simulink model "UKFSIM"  (R2019a)
settings: Solver=VariableStepAuto  StartTime=0.0  StopTime=50000  RelTol=1e-3
values from neighbouring files (symbols this model uses):
  A1 = 5    [run.m]
  A2 = 5    [run.m]
  A3 = 5    [run.m]
libraries: simulink x1
settings Model: Creator=Nima  LastModifiedBy=Nima

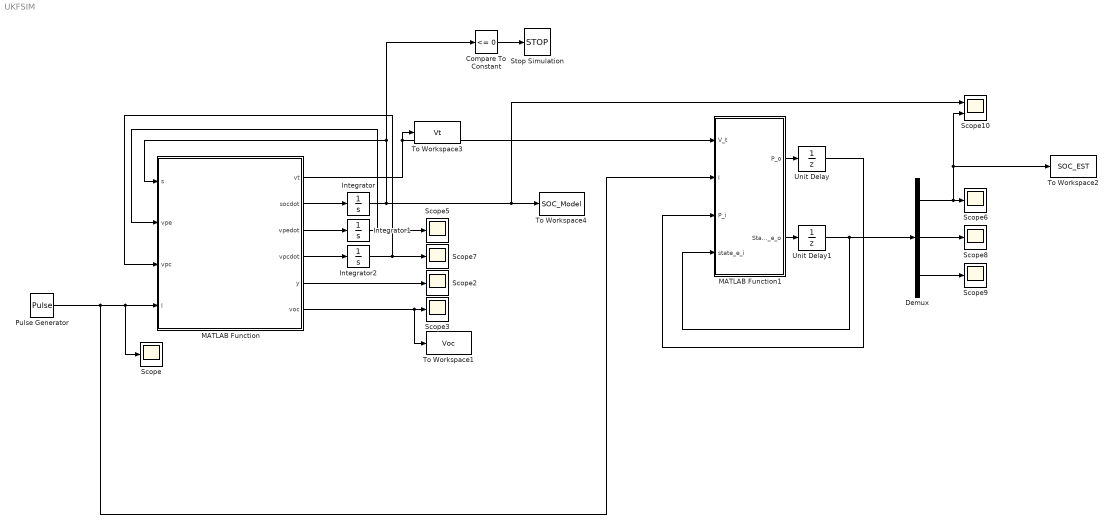
== system UKFSIM ==
  Compare To Constant : simulink/Logic and Bit Operations/Compare To Constant  relop=<=  const=0  OutDataTypeStr=boolean
  Demux : Demux  Outputs=3
  Integrator : Integrator  InitialCondition=1
  Integrator1 : Integrator
  Integrator2 : Integrator
  MATLAB Function : MATLAB Function  TreatAsAtomicUnit=on
  MATLAB Function1 : MATLAB Function  TreatAsAtomicUnit=on
  Pulse Generator : DiscretePulseGenerator  PulseType=Time based  Amplitude=5  Period=5000  PulseWidth=10
  Scope{,2..3,5..9} (8 alike) : Scope
  Scope10 : Scope  NumInputPorts=2
  Stop Simulation : Stop
  To Workspace1 : ToWorkspace  VariableName=Voc  SaveFormat=Timeseries  SampleTime=-1
  To Workspace2 : ToWorkspace  VariableName=SOC_EST  SaveFormat=Timeseries  SampleTime=-1
  To Workspace3 : ToWorkspace  VariableName=Vt  SaveFormat=Timeseries  SampleTime=-1
  To Workspace4 : ToWorkspace  VariableName=SOC_Model  SaveFormat=Timeseries  SampleTime=-1
  Unit Delay : UnitDelay  InitialCondition=diag([A1 A2 A3])  SampleTime=0.01  HasFrameUpgradeWarning=on
  Unit Delay1 : UnitDelay  InitialCondition=[0.2,0,0]  SampleTime=0.01  HasFrameUpgradeWarning=on
  wires:
  MATLAB Function/2(socdot) -> Integrator/1
  MATLAB Function/3(vpedot) -> Integrator1/1
  MATLAB Function/4(vpcdot) -> Integrator2/1
  MATLAB Function/5(y) -> Scope2/1
  MATLAB Function/6(voc) -> To Workspace1/1, Scope3/1
  Integrator1/1 -> MATLAB Function/2(vpe), Scope5/1
  Unit Delay1/1 -> Demux/1, MATLAB Function1/4(state_e_i)
  MATLAB Function/1(vt) -> MATLAB Function1/1(V_t), To Workspace3/1
  MATLAB Function1/1(P_o) -> Unit Delay/1
  MATLAB Function1/2(State_e_o) -> Unit Delay1/1
  Pulse Generator/1 -> MATLAB Function1/2(I), Scope/1, MATLAB Function/4(I)
  Unit Delay/1 -> MATLAB Function1/3(P_i)
  Demux/2 -> Scope8/1
  Demux/1 -> To Workspace2/1, Scope10/2, Scope6/1
  Demux/3 -> Scope9/1
  Compare To Constant/1 -> Stop Simulation/1
  Integrator/1 -> Scope10/1, To Workspace4/1, Compare To Constant/1, MATLAB Function/1(s)
  Integrator2/1 -> MATLAB Function/3(vpc), Scope7/1

== matlab function UKFSIM/MATLAB Function1 ==
  data: V_t input; P_o output; I input; P_i input; state_e_i input; State_e_o output
function [P_o,State_e_o] = fcn(V_t,I,P_i,state_e_i)
%%
%{
sigma_xx(:,k)=[
    sigma_x(1,k)=soc(k-1);
    sigma_x(2,k)=Vpe(k-1);
    sigma_x(3,k)=Vpc(k-1);
]

sigma_xxx(:,i)-->
sigma_xxx(1,k)= soc(k-1);
sigma_xxx(2,k)= Vpe(k-1);
sigma_xxx(3,k)= Vpc(k-1);
sigma_z(1,k)=vt;
%}
%% Battery Parameters
R_pe=4.96e-3;
R_pc=2.86e-3;
C_pe=4.93e3;
C_pc=14.33e3;
R_in=102.5e-3;
C_n=5*3600;
%% 
n=3;
n_m=2*n+1;
kappa=0;
alpha=0.6;
beta=300;
%% 7.34
lambda=alpha^2*(n+kappa)-n;
wm = ones(n_m,1)*1/(2*(n+lambda));
wc = wm;
wm(1)= lambda/(lambda+n); 
wc(1)= lambda/(lambda+n)+1-alpha^2+beta;
sigma_x=zeros(3,n_m);
sigma_xx=zeros(3,n_m);
sigma_xxx=zeros(3,n_m);
sigma_z=zeros(1,n_m);
P_sqrt=chol(P_i,'lower');
%%
% Q = diag([0.02 0.1 0.2]);R=0.2;   
%% 7.39 Calculate sigma point
for i=1:1:n_m
    if i==1
        sigma_x(:,i)= state_e_i;
    elseif i>=2 && i<=n+1
        sigma_x(:,i)= state_e_i+sqrt(n+lambda)*(P_sqrt(:,i-1));
    elseif i>n+1
        sigma_x(:,i)= state_e_i-sqrt(n+lambda)*(P_sqrt(:,i-1-n));
    end
end
%% Time Update 7.41
for k=1:1:n_m 
    sigma_xx(:,k)=[sigma_x(1,k)-0.01*(I/C_n);
                   sigma_x(2,k)+0.01*((-1/(R_pe*C_pe))*sigma_x(2,k)+I/C_pe);
                   sigma_x(3,k)+0.01*((-1/(R_pc*C_pc))*sigma_x(3,k)+I/C_pe)
                   ];
end
%% 7.41
x_n=sigma_xx*wm;
P_n=zeros(3,3);
%% 7.42
for k=1:n_m
    P_n=P_n+wc(k)*(sigma_xx(:,k)-x_n)*(sigma_xx(:,k)-x_n)'  ;
end

P_sqrt=chol(P_n,'lower');
%% 7.39 Calculate sigma point
for i=1:1:n_m
    if i==1
        sigma_xxx(:,i)= x_n;
    elseif i>=2 && i<=n+1
        sigma_xxx(:,i)= x_n+sqrt(n+lambda)*(P_sqrt(:,i-1));
    elseif i>n+1
        sigma_xxx(:,i)= x_n-sqrt(n+lambda)*(P_sqrt(:,i-1-n));
    end
end

%% Time Update 
for k=1:1:n_m
% V_oc=3.608-1.209*sigma_xxx(1,k)^4 + 3.055*sigma_xxx(1,k)^3 - 2.215*sigma_xxx(1,k)^2 +0.9301*sigma_xxx(1,k);
V_oc=0.55*sigma_xxx(1,k)+3.625;
sigma_z(:,k)=V_oc-sigma_xxx(2,k)-sigma_xxx(3,k)-I*R_in;
end
z_n=sigma_z*wm;
%% Measurement update equations
Pyy=10^-5;
Pxy=zeros(n,1);
%% 7.45 , 7.46
for k=1:1:n_m
    Pyy=Pyy+wc(k)*(sigma_z(:,k)-z_n)*(sigma_z(:,k)-z_n)'  ;
    Pxy=Pxy+wc(k)*(sigma_xxx(:,k)-x_n)*(sigma_z(:,k)-z_n)';
end
%% 7.47-49
K=Pxy/Pyy;
State_e_o=x_n+K*(V_t-z_n);
P_o=P_n-K*Pyy*K';

== matlab function UKFSIM/MATLAB Function ==
  data: s input; vpe input; vpc input; I input; vt output; socdot output; vpedot output; vpcdot output; y output; voc output
function [vt,socdot,vpedot,vpcdot,y,voc]  = fcn(s,vpe,vpc,I)
%% Battery Parameters
Rpe=4.96e-3;
Rpc=2.86e-3;
Cpe=4.93e3;
Cpc=14.33e3;
Rin=102.5e-3;
Cn=5*3600;
k=0.55;
%%
a1 = 1/(Rpe*Cpe)+1/(Rpc*Cpc);
a2 = 1/(Rin*Cn);
a3 = 1/(Rpc*Cpc);
a4 = 1/(Rpe*Cpe);
b1 = k/Cn + 1/Cpe + 1/Cpc + Rin/(Rpe*Cpe)+ Rin/(Rpc*Cpc);
b2 = 1/Cpe;
b3 = 1/Cpc;
% uncer=0.2;
%%
voc=k*s+3.625;
% voc=3.608-1.209*s^4 + 3.055*s^3 - 2.215*s^2 +0.9301*s;
vt=voc-vpe-vpc-Rin*I;
socdot=a2*vt - a2*(voc) + a2*vpc + a2*vpe;%-0.0326*uncer;
vpedot=-a4*vpe + b2*I;%+0.0122*uncer;
vpcdot=-a3*vpc+b3*I;%+0.0204*uncer;
y=vt;
% %% State Space Modeling
% x=[x1;x2;x3];
% A=[-a1  a1  0;
%     a2 -a2  -a2;
%     0    0  -a1];
% z=a3+a4+a5;
% C=[1 0 0];
% B=[z;0;a4];
% %% SOC
% p1 = 0.0173;  
% p2 = -0.7373; 
% p3= 7.855;
% % SOC = p1*ocv^2 + p2*ocv + p3;
% 
% %% Output
% Xdot=A*x+B*u;
% Yt=C*x;
% soc = p1*x2^2 + p2*x2 + p3;
